simulink model "ModeAdjust"  (R2018b)
settings: Solver=FixedStepDiscrete  StartTime=0.0  StopTime=inf  FixedStep=0.01  RelTol=1e-3
undefined symbols (not defined in the file or in its folder): IfKeSMSbSeatMovBkRclnEnable_Val, IfKeSMSbSeatMovFrwdBkwdEnable_Val, IfKeSMSbSeatMovFtrstEnable_Val, IfKeSMSbSeatMovHdrstFrwdBkwdEnable_Val, IfKeSMSbSeatMovHdUpwdDnwdEnable_Val, IfKeSMSbSeatMovLgrstEnable_Val, IfKeSMSbSeatMovLtwdRtwdEnable_Val, IfVeSMSeStNumConfig, KeSMSbArmscreenMovEnable_Val, KeSMSbSeatMovLgrstExpdEnable_Val, KeSMSuFirstRwStBackPosDelta_Val, KeSMSuFirstRwStBackPosTolr_Val, KeSMSuFirstRwStCushFrntPosDelta_Val, KeSMSuFirstRwStCushFrntPosTolr_Val, KeSMSuFirstRwStCushRePosDelta_Val, KeSMSuFirstRwStCushRePosTolr_Val, KeSMSuFirstRwStFootrestPosDelta_Val, KeSMSuFirstRwStFootrestPosTolr_Val, KeSMSuFirstRwStFwdBkwdPosDelta_Val, KeSMSuFirstRwStFwdBkwdPosTolr_Val, KeSMSuMdMotFinshdTm_Val, KeSMSuMdRetryTm1_Val, KeSMSuModeReqDurgTm_Val, KeSMSuSecRwStArmTochPosDelta_Val, KeSMSuSecRwStArmTochPosTolr_Val, KeSMSuSecRwStBackPosDelta_Val, KeSMSuSecRwStBackPosTolr_Val, KeSMSuSecRwStFtrstUpwdDnwdPosDelta_Val, KeSMSuSecRwStFtrstUpwdDnwdPosTolr_Val, KeSMSuSecRwStFwdBkwdPosDelta_Val, KeSMSuSecRwStFwdBkwdPosTolr_Val, KeSMSuSecRwStHeadrestFwdBkwdPosDelta_Val, KeSMSuSecRwStHeadrestFwdBkwdPosTolr_Val, KeSMSuSecRwStHeadrestUpwdDwnwdPosDelta_Val, KeSMSuSecRwStHeadrestUpwdDwnwdPosTolr_Val, KeSMSuSecRwStLegrestInOutPosDelta_Val, KeSMSuSecRwStLegrestInOutPosTolr_Val, KeSMSuSecRwStLegrestUpwdDwnwdPosDelta_Val, KeSMSuSecRwStLegrestUpwdDwnwdPosTolr_Val, KeSMSuSecRwStLwdRwdPosDelta_Val, KeSMSuSecRwStLwdRwdPosTolr_Val, KeSMSuSecRwStVIPFtrstRefAngle_Val, KeSMSuThirdRwStFwdBkwdPosDelta_Val, KeSMSuThirdRwStFwdBkwdPosTolr_Val, KeSMSuThrdRwCushFoldPosDelta_Val, KeSMSuThrdRwCushFoldPosTolr_Val, KeSMSuThrdRwStBackPosDelta_Val, KeSMSuThrdRwStBackPosTolr_Val, KeSMSw4SLegrstCloseMdSecRwLtStFtrstUpwdDnwdPos_Val, KeSMSw4SLegrstCloseMdSecRwLtStFtrstUpwdDnwdPosMax_Val, KeSMSw4SLegrstCloseMdSecRwLtStFtrstUpwdDnwdPosMin_Val, KeSMSw4SLegrstCloseMdSecRwLtStLgrstOtwdInwdPos_Val, KeSMSw4SLegrstCloseMdSecRwLtStLgrstOtwdInwdPosMax_Val, KeSMSw4SLegrstCloseMdSecRwLtStLgrstOtwdInwdPosMin_Val, KeSMSw4SLegrstCloseMdSecRwLtStLgrstUpwdDnwdPos_Val, KeSMSw4SLegrstCloseMdSecRwLtStLgrstUpwdDnwdPosMax_Val, KeSMSw4SLegrstCloseMdSecRwLtStLgrstUpwdDnwdPosMin_Val, KeSMSw4SLegrstCloseMdSecRwRtStFtrstUpwdDnwdPos_Val, KeSMSw4SLegrstCloseMdSecRwRtStFtrstUpwdDnwdPosMax_Val, KeSMSw4SLegrstCloseMdSecRwRtStFtrstUpwdDnwdPosMin_Val ... (+1138)
libraries: Lib x401
(part 32 of 35)

== system ModeAdjust/ModeAdjustRunnable_sys/ModeAdjust/ArrivedAtTargetPosChk/VIP/R2Rt ==
  SecRwRtStPoss : Inport
  ModeStCalib_2R : Inport  Port=2
  StConfig : Inport  Port=3
  SecRwRtStPossV : Inport  Port=4
  PosDeltaCalib : Inport  Port=5
  Bus Selector : BusSelector  OutputSignals=IfVeSMSuSecRwRtStBkReclnUpwdDnwdPos_Val_read,IfVeSMSuSecRwRtStFrwdBkwdPos_Val_read,IfVeSMSuSecRwRtStHPassStUpwdDnwdPos_Val_read,IfVeSMSuSecRwRtStLgrstUpwdDnwdPos_Val_read,IfVeSMSuSecRwRtStLtwdRtwdPos_Val_read,SecRwRtStArmScrnPos_Val_read
  Bus Selector1 : BusSelector  OutputSignals=IfVeSMSuSecRwRtStBkReclnUpwdDnwdPosV_Val_read,IfVeSMSuSecRwRtStFrwdBkwdPosV_Val_read,IfVeSMSuSecRwRtStHPassStUpwdDnwdPosV_Val_read,IfVeSMSuSecRwRtStLgrstUpwdDnwdPosV_Val_read,IfVeSMSuSecRwRtStLtwdRtwdPosV_Val_read,SecRwRtStArmScrnPosV_Val_read
  Bus Selector2 : BusSelector  OutputSignals=ArmScrnPos,ArmScrnPosMax,ArmScrnPosMin,BkReclnUpwdDnwdPos,BkReclnUpwdDnwdPosMax,BkReclnUpwdDnwdPosMin,FrwdBkwdPos,FrwdBkwdPosMax,FrwdBkwdPosMin,HdrstUpwdPos,HdrstUpwdPosMax,HdrstUpwdPosMin,LgrstUpwdPos,LgrstUpwdPosMax,LgrstUpwdPosMin,LtwdRtwdPos,LtwdRtwdPosMax,LtwdRtwdPosMin
  Bus Selector3 : BusSelector  OutputSignals=VIPSecRwRtSt
  Bus Selector4 : BusSelector  OutputSignals=BkReclnUpwdDnwdMovConfig,ArmTouchMovConfig,FrwdBkwdMovConfig,LgrstUpwdMovConfig,LtwdRtwdMovConfig
  Bus Selector5 : BusSelector  OutputSignals=KeSMSuSecRwStArmTochPosDelta_Val,KeSMSuSecRwStBackPosDelta_Val,KeSMSuSecRwStFwdBkwdPosDelta_Val,KeSMSuSecRwStLegrestUpwdDwnwdPosDelta_Val,KeSMSuSecRwStLwdRwdPosDelta_Val
  CheckAtPos{,1..3} (4 alike) : Lib/CheckAtPos  SystemSampleTime=-1
  Constant{1..8} (8 alike) : Constant  Value=0  OutDataTypeStr=boolean
  IsArrivedTarZone{,1,3..4} (4 alike) : Lib/CommonUsed/IniPosjudg/Subsystem2  SystemSampleTime=-1
  Logical Operator9 : Logic  Inputs=4  AllPortsSameDT=off  OutDataTypeStr=boolean
  R2Rt_ArrivedTarPos : Outport
  wires:
  Logical Operator9/1 -> R2Rt_ArrivedTarPos/1
  IsArrivedTarZone4/1 -> [Step2_2_ArrivedTarPos]
  [SecRwRtStLtwdRtwdPos] -> IsArrivedTarZone4/1
  Bus Selector/2 -> [SecRwRtStFrwdBkwdPos]  "<IfVeSMSuSecRwRtStFrwdBkwdPos_Val_read>"
  Bus Selector/3 -> [SecRwRtStHPassStUpwdDnwdPos]  "<IfVeSMSuSecRwRtStHPassStUpwdDnwdPos_Val_read>"
  SecRwRtStPoss/1 -> Bus Selector/1
  Bus Selector/5 -> [SecRwRtStLtwdRtwdPos]  "<IfVeSMSuSecRwRtStLtwdRtwdPos_Val_read>"
  Bus Selector/1 -> [SecRwRtStBkReclnUpwdDnwdPos]  "<IfVeSMSuSecRwRtStBkReclnUpwdDnwdPos_Val_read>"
  Bus Selector/4 -> [SecRwRtStLgrstUpwdDnwdPos]  "<IfVeSMSuSecRwRtStLgrstUpwdDnwdPos_Val_read>"
  [SecRwRtStFrwdBkwdPos] -> IsArrivedTarZone3/1
  IsArrivedTarZone3/1 -> [Step2_1_ArrivedTarPos]
  IsArrivedTarZone/1 -> [Step1_1_ArrivedTarPos]
  [SecRwRtStBkReclnUpwdDnwdPos] -> IsArrivedTarZone/1
  [K_BkReclnUpwdDnwdPosMin] -> IsArrivedTarZone/2
  [K_FrwdBkwdPosMin] -> IsArrivedTarZone3/2
  [K_LgrstUpwdPosMin] -> IsArrivedTarZone1/2
  [SecRwRtStLgrstUpwdDnwdPos] -> IsArrivedTarZone1/1
  IsArrivedTarZone1/1 -> [Step1_2_ArrivedTarPos]
  Bus Selector/6 -> [SecRwRtStArmScrnPos]  "<SecRwRtStArmScrnPos_Val_read>"
  [K_LtwdRtwdPosMin] -> IsArrivedTarZone4/2
  [KeSMSuSecRwStBackPosDelta_Val] -> IsArrivedTarZone/3
  [KeSMSuSecRwStLegrestUpwdDwnwdPosDelta_Val] -> IsArrivedTarZone1/3
  [KeSMSuSecRwStFwdBkwdPosDelta_Val] -> IsArrivedTarZone3/3
  [KeSMSuSecRwStLwdRwdPosDelta_Val] -> IsArrivedTarZone4/3
  [K_BkReclnUpwdDnwdPosMax] -> IsArrivedTarZone/4
  [K_LgrstUpwdPosMax] -> IsArrivedTarZone1/4
  [K_FrwdBkwdPosMax] -> IsArrivedTarZone3/4
  [K_LtwdRtwdPosMax] -> IsArrivedTarZone4/4
  Bus Selector2/1 -> [K_ArmScrnPos]  "<ArmScrnPos>"
  Bus Selector2/18 -> [K_LtwdRtwdPosMin]  "<LtwdRtwdPosMin>"
  Bus Selector2/16 -> [K_LtwdRtwdPos]  "<LtwdRtwdPos>"
  Bus Selector2/15 -> [K_LgrstUpwdPosMin]  "<LgrstUpwdPosMin>"
  Bus Selector2/17 -> [K_LtwdRtwdPosMax]  "<LtwdRtwdPosMax>"
  Bus Selector2/12 -> [K_HdrstUpwdPosMin]  "<HdrstUpwdPosMin>"
  Bus Selector2/13 -> [K_LgrstUpwdPos]  "<LgrstUpwdPos>"
  Bus Selector2/11 -> [K_HdrstUpwdPosMax]  "<HdrstUpwdPosMax>"
  Bus Selector2/14 -> [K_LgrstUpwdPosMax]  "<LgrstUpwdPosMax>"
  Bus Selector2/10 -> [K_HdrstUpwdPos]  "<HdrstUpwdPos>"
  Bus Selector2/4 -> [K_BkReclnUpwdDnwdPos]  "<BkReclnUpwdDnwdPos>"
  Bus Selector2/9 -> [K_FrwdBkwdPosMin]  "<FrwdBkwdPosMin>"
  Bus Selector2/5 -> [K_BkReclnUpwdDnwdPosMax]  "<BkReclnUpwdDnwdPosMax>"
  Bus Selector2/8 -> [K_FrwdBkwdPosMax]  "<FrwdBkwdPosMax>"
  Bus Selector3/1 -> Bus Selector2/1  "<VIPSecRwRtSt>"
  Bus Selector2/7 -> [K_FrwdBkwdPos]  "<FrwdBkwdPos>"
  Bus Selector2/3 -> [K_ArmScrnPosMin]  "<ArmScrnPosMin>"
  Bus Selector2/2 -> [K_ArmScrnPosMax]  "<ArmScrnPosMax>"
  Bus Selector2/6 -> [K_BkReclnUpwdDnwdPosMin]  "<BkReclnUpwdDnwdPosMin>"
  ModeStCalib_2R/1 -> Bus Selector3/1
  StConfig/1 -> Bus Selector4/1
  Bus Selector4/3 -> [FrwdBkwdMovConfig]  "<FrwdBkwdMovConfig>"
  Bus Selector4/5 -> [LtwdRtwdMovConfig]  "<LtwdRtwdMovConfig>"
  Bus Selector4/4 -> [LgrstUpwdMovConfig]  "<LgrstUpwdMovConfig>"
  Bus Selector4/2 -> [ArmTouchMovConfig]  "<ArmTouchMovConfig>"
  Bus Selector4/1 -> [BkReclnUpwdDnwdMovConfig]  "<BkReclnUpwdDnwdMovConfig>"
  Bus Selector1/1 -> [SecRwRtStBkReclnUpwdDnwdPosV]  "<IfVeSMSuSecRwRtStBkReclnUpwdDnwdPosV_Val_read>"
  Bus Selector1/5 -> [SecRwRtStLtwdRtwdPosV]  "<IfVeSMSuSecRwRtStLtwdRtwdPosV_Val_read>"
  Bus Selector1/4 -> [SecRwRtStLgrstUpwdDnwdPosV]  "<IfVeSMSuSecRwRtStLgrstUpwdDnwdPosV_Val_read>"
  Bus Selector1/6 -> [SecRwRtStArmScrnPosV]  "<SecRwRtStArmScrnPosV_Val_read>"
  SecRwRtStPossV/1 -> Bus Selector1/1
  Bus Selector1/3 -> [SecRwRtStHPassStUpwdDnwdPosV]  "<IfVeSMSuSecRwRtStHPassStUpwdDnwdPosV_Val_read>"
  Bus Selector1/2 -> [SecRwRtStFrwdBkwdPosV]  "<IfVeSMSuSecRwRtStFrwdBkwdPosV_Val_read>"
  CheckAtPos2/1 -> Logical Operator9/3  "VIPR_Step2_1_ArrivedTarPos"
  CheckAtPos3/1 -> Logical Operator9/4  "VIPR_Step2_2_ArrivedTarPos"
  CheckAtPos1/1 -> Logical Operator9/2  "VIPR_Step1_2_ArrivedTarPos"
  CheckAtPos/1 -> Logical Operator9/1  "VIPR_Step1_1_ArrivedTarPos"
  [BkReclnUpwdDnwdMovConfig] -> CheckAtPos/1
  [Step1_1_ArrivedTarPos] -> CheckAtPos/3
  [LgrstUpwdMovConfig] -> CheckAtPos1/1
  [Step1_2_ArrivedTarPos] -> CheckAtPos1/3
  [FrwdBkwdMovConfig] -> CheckAtPos2/1
  [Step2_1_ArrivedTarPos] -> CheckAtPos2/3
  [LtwdRtwdMovConfig] -> CheckAtPos3/1
  [Step2_2_ArrivedTarPos] -> CheckAtPos3/3
  [SecRwRtStBkReclnUpwdDnwdPosV] -> CheckAtPos/2
  [SecRwRtStFrwdBkwdPosV] -> CheckAtPos2/2
  [SecRwRtStLgrstUpwdDnwdPosV] -> CheckAtPos1/2
  [SecRwRtStLtwdRtwdPosV] -> CheckAtPos3/2
  Constant3/1 -> CheckAtPos3/5
  Constant2/1 -> CheckAtPos3/4
  Constant4/1 -> CheckAtPos2/5
  Constant1/1 -> CheckAtPos2/4
  Constant6/1 -> CheckAtPos1/5
  Constant5/1 -> CheckAtPos1/4
  Constant8/1 -> CheckAtPos/5
  Constant7/1 -> CheckAtPos/4
  Bus Selector5/5 -> [KeSMSuSecRwStLwdRwdPosDelta_Val]  "<KeSMSuSecRwStLwdRwdPosDelta_Val>"
  PosDeltaCalib/1 -> Bus Selector5/1
  Bus Selector5/2 -> [KeSMSuSecRwStBackPosDelta_Val]  "<KeSMSuSecRwStBackPosDelta_Val>"
  Bus Selector5/4 -> [KeSMSuSecRwStLegrestUpwdDwnwdPosDelta_Val]  "<KeSMSuSecRwStLegrestUpwdDwnwdPosDelta_Val>"
  Bus Selector5/1 -> [KeSMSuSecRwStArmTochPosDelta_Val]  "<KeSMSuSecRwStArmTochPosDelta_Val>"
  Bus Selector5/3 -> [KeSMSuSecRwStFwdBkwdPosDelta_Val]  "<KeSMSuSecRwStFwdBkwdPosDelta_Val>"

== system ModeAdjust/ModeAdjustRunnable_sys/ModeAdjust/ArrivedAtTargetPosChk/VIP/R3Lt ==
  ThdRwLtStPoss : Inport
  ModeStCalib_3L : Inport  Port=2
  StConfig : Inport  Port=3
  ThdRwLtStPossV : Inport  Port=4
  PosDeltaCalib : Inport  Port=5
  Bus Selector : BusSelector  OutputSignals=IfVeSMSuThdRwLtStBkReclnUpwdDnwdPos_Val_read,IfVeSMSuThdRwLtStCshnFldUpwdDnwdPos_Val_read,IfVeSMSuThdRwLtStFrwdBkwdPos_Val_read
  Bus Selector1 : BusSelector  OutputSignals=IfVeSMSuThdRwLtStBkReclnUpwdDnwdPosV_Val_read,IfVeSMSuThdRwLtStCshnFldUpwdDnwdPosV_Val_read,IfVeSMSuThdRwLtStFrwdBkwdPosV_Val_read
  Bus Selector2 : BusSelector  OutputSignals=BkReclnUpwdDnwdPos,BkReclnUpwdDnwdPosMax,BkReclnUpwdDnwdPosMin,CshnFldUpwdDnwdPos,CshnFldUpwdDnwdPosMax,CshnFldUpwdDnwdPosMin,FrwdBkwdPos,FrwdBkwdPosMax,FrwdBkwdPosMin
  Bus Selector3 : BusSelector  OutputSignals=VIPThdRwLtSt
  Bus Selector4 : BusSelector  OutputSignals=BkReclnUpwdDnwdMovConfig,CshnFldUpwdDnwdMovConfig,FrwdBkwdMovConfig
  Bus Selector5 : BusSelector  OutputSignals=KeSMSuThirdRwStFwdBkwdPosDelta_Val,KeSMSuThrdRwCushFoldPosDelta_Val,KeSMSuThrdRwStBackPosDelta_Val
  CheckAtPos : Lib/CheckAtPos  SystemSampleTime=-1
  CheckAtPos1 : Lib/CheckAtPos  SystemSampleTime=-1
  Constant{1..4} (4 alike) : Constant  Value=0  OutDataTypeStr=boolean
  IsArrivedTarZone : Lib/CommonUsed/IniPosjudg/Subsystem2  SystemSampleTime=-1
  IsArrivedTarZone1 : Lib/CommonUsed/IniPosjudg/Subsystem2  SystemSampleTime=-1
  Logical Operator3 : Logic  AllPortsSameDT=off  OutDataTypeStr=boolean
  R3Lt_ArrivedTarPos : Outport
  wires:
  Logical Operator3/1 -> R3Lt_ArrivedTarPos/1
  Bus Selector/1 -> [ThdRwLtStBkReclnUpwdDnwdPos]  "<IfVeSMSuThdRwLtStBkReclnUpwdDnwdPos_Val_read>"
  Bus Selector/3 -> [ThdRwLtStFrwdBkwdPos]  "<IfVeSMSuThdRwLtStFrwdBkwdPos_Val_read>"
  ThdRwLtStPoss/1 -> Bus Selector/1
  Bus Selector/2 -> [ThdRwLtStCshnFldUpwdDnwdPos]  "<IfVeSMSuThdRwLtStCshnFldUpwdDnwdPos_Val_read>"
  [ThdRwLtStFrwdBkwdPos] -> IsArrivedTarZone1/1
  IsArrivedTarZone1/1 -> [Step2ArrivedTarPos]
  IsArrivedTarZone/1 -> [Step1ArrivedTarPos]
  [ThdRwLtStBkReclnUpwdDnwdPos] -> IsArrivedTarZone/1
  [K_BkReclnUpwdDnwdPosMin] -> IsArrivedTarZone/2
  [K_FrwdBkwdPosMin] -> IsArrivedTarZone1/2
  [K_BkReclnUpwdDnwdPosMax] -> IsArrivedTarZone/4
  [KeSMSuThrdRwStBackPosDelta_Val] -> IsArrivedTarZone/3
  [KeSMSuThirdRwStFwdBkwdPosDelta_Val] -> IsArrivedTarZone1/3
  [K_FrwdBkwdPosMax] -> IsArrivedTarZone1/4
  Bus Selector2/6 -> [K_CshnFldUpwdDnwdPosMin]  "<CshnFldUpwdDnwdPosMin>"
  Bus Selector2/4 -> [K_CshnFldUpwdDnwdPos]  "<CshnFldUpwdDnwdPos>"
  Bus Selector2/7 -> [K_FrwdBkwdPos]  "<FrwdBkwdPos>"
  Bus Selector2/5 -> [K_CshnFldUpwdDnwdPosMax]  "<CshnFldUpwdDnwdPosMax>"
  ModeStCalib_3L/1 -> Bus Selector3/1
  Bus Selector2/3 -> [K_BkReclnUpwdDnwdPosMin]  "<BkReclnUpwdDnwdPosMin>"
  Bus Selector3/1 -> Bus Selector2/1  "<VIPThdRwLtSt>"
  Bus Selector2/9 -> [K_FrwdBkwdPosMin]  "<FrwdBkwdPosMin>"
  Bus Selector2/2 -> [K_BkReclnUpwdDnwdPosMax]  "<BkReclnUpwdDnwdPosMax>"
  Bus Selector2/1 -> [K_BkReclnUpwdDnwdPos]  "<BkReclnUpwdDnwdPos>"
  Bus Selector2/8 -> [K_FrwdBkwdPosMax]  "<FrwdBkwdPosMax>"
  Bus Selector4/1 -> [BkReclnUpwdDnwdMovConfig]  "<BkReclnUpwdDnwdMovConfig>"
  StConfig/1 -> Bus Selector4/1
  Bus Selector4/2 -> [CshnFldUpwdDnwdMovConfig]  "<CshnFldUpwdDnwdMovConfig>"
  Bus Selector4/3 -> [FrwdBkwdMovConfig]  "<FrwdBkwdMovConfig>"
  ThdRwLtStPossV/1 -> Bus Selector1/1
  Bus Selector1/3 -> [ThdRwLtStFrwdBkwdPosV]  "<IfVeSMSuThdRwLtStFrwdBkwdPosV_Val_read>"
  Bus Selector1/2 -> [ThdRwLtStCshnFldUpwdDnwdPosV]  "<IfVeSMSuThdRwLtStCshnFldUpwdDnwdPosV_Val_read>"
  Bus Selector1/1 -> [ThdRwLtStBkReclnUpwdDnwdPosV]  "<IfVeSMSuThdRwLtStBkReclnUpwdDnwdPosV_Val_read>"
  CheckAtPos/1 -> Logical Operator3/1
  CheckAtPos1/1 -> Logical Operator3/2
  [BkReclnUpwdDnwdMovConfig] -> CheckAtPos/1
  [Step1ArrivedTarPos] -> CheckAtPos/3
  [FrwdBkwdMovConfig] -> CheckAtPos1/1
  [Step2ArrivedTarPos] -> CheckAtPos1/3
  [ThdRwLtStBkReclnUpwdDnwdPosV] -> CheckAtPos/2
  [ThdRwLtStFrwdBkwdPosV] -> CheckAtPos1/2
  Constant3/1 -> CheckAtPos/5
  Constant2/1 -> CheckAtPos/4
  Constant4/1 -> CheckAtPos1/5
  Constant1/1 -> CheckAtPos1/4
  PosDeltaCalib/1 -> Bus Selector5/1
  Bus Selector5/2 -> [KeSMSuThrdRwCushFoldPosDelta_Val]  "<KeSMSuThrdRwCushFoldPosDelta_Val>"
  Bus Selector5/1 -> [KeSMSuThirdRwStFwdBkwdPosDelta_Val]  "<KeSMSuThirdRwStFwdBkwdPosDelta_Val>"
  Bus Selector5/3 -> [KeSMSuThrdRwStBackPosDelta_Val]  "<KeSMSuThrdRwStBackPosDelta_Val>"

== system ModeAdjust/ModeAdjustRunnable_sys/ModeAdjust/ArrivedAtTargetPosChk/VIP/R3Rt ==
  ThdRwRtStPoss : Inport
  ModeStCalib_3R : Inport  Port=2
  StConfig : Inport  Port=3
  ThdRwRtStPossV : Inport  Port=4
  PosDeltaCalib : Inport  Port=5
  Bus Selector : BusSelector  OutputSignals=IfVeSMSuThdRwRtStBkReclnUpwdDnwdPos_Val_read,IfVeSMSuThdRwRtStCshnFldUpwdDnwdPos_Val_read,IfVeSMSuThdRwRtStFrwdBkwdPos_Val_read
  Bus Selector1 : BusSelector  OutputSignals=IfVeSMSuThdRwRtStBkReclnUpwdDnwdPosV_Val_read,IfVeSMSuThdRwRtStCshnFldUpwdDnwdPosV_Val_read,IfVeSMSuThdRwRtStFrwdBkwdPosV_Val_read
  Bus Selector2 : BusSelector  OutputSignals=BkReclnUpwdDnwdPos,BkReclnUpwdDnwdPosMax,BkReclnUpwdDnwdPosMin,CshnFldUpwdDnwdPos,CshnFldUpwdDnwdPosMax,CshnFldUpwdDnwdPosMin,FrwdBkwdPos,FrwdBkwdPosMax,FrwdBkwdPosMin
  Bus Selector3 : BusSelector  OutputSignals=VIPThdRwRtSt
  Bus Selector4 : BusSelector  OutputSignals=BkReclnUpwdDnwdMovConfig,CshnFldUpwdDnwdMovConfig,FrwdBkwdMovConfig
  Bus Selector5 : BusSelector  OutputSignals=KeSMSuThirdRwStFwdBkwdPosDelta_Val,KeSMSuThrdRwCushFoldPosDelta_Val,KeSMSuThrdRwStBackPosDelta_Val
  CheckAtPos : Lib/CheckAtPos  SystemSampleTime=-1
  CheckAtPos1 : Lib/CheckAtPos  SystemSampleTime=-1
  Constant{1..4} (4 alike) : Constant  Value=0  OutDataTypeStr=boolean
  IsArrivedTarZone : Lib/CommonUsed/IniPosjudg/Subsystem2  SystemSampleTime=-1
  IsArrivedTarZone1 : Lib/CommonUsed/IniPosjudg/Subsystem2  SystemSampleTime=-1
  Logical Operator3 : Logic  AllPortsSameDT=off  OutDataTypeStr=boolean
  R3Rt_ArrivedTarPos : Outport
  wires:
  Logical Operator3/1 -> R3Rt_ArrivedTarPos/1
  Bus Selector/1 -> [ThdRwRtStBkReclnUpwdDnwdPos]  "<IfVeSMSuThdRwRtStBkReclnUpwdDnwdPos_Val_read>"
  Bus Selector/2 -> [ThdRwRtStCshnFldUpwdDnwdPos]  "<IfVeSMSuThdRwRtStCshnFldUpwdDnwdPos_Val_read>"
  ThdRwRtStPoss/1 -> Bus Selector/1
  Bus Selector/3 -> [ThdRwRtStFrwdBkwdPos]  "<IfVeSMSuThdRwRtStFrwdBkwdPos_Val_read>"
  [K_FrwdBkwdPosMin] -> IsArrivedTarZone1/2
  [K_BkReclnUpwdDnwdPosMin] -> IsArrivedTarZone/2
  [ThdRwRtStBkReclnUpwdDnwdPos] -> IsArrivedTarZone/1
  IsArrivedTarZone/1 -> [Step1ArrivedTarPos]
  IsArrivedTarZone1/1 -> [Step2ArrivedTarPos]
  [ThdRwRtStFrwdBkwdPos] -> IsArrivedTarZone1/1
  [KeSMSuThrdRwStBackPosDelta_Val] -> IsArrivedTarZone/3
  [KeSMSuThirdRwStFwdBkwdPosDelta_Val] -> IsArrivedTarZone1/3
  [K_BkReclnUpwdDnwdPosMax] -> IsArrivedTarZone/4
  [K_FrwdBkwdPosMax] -> IsArrivedTarZone1/4
  Bus Selector2/6 -> [K_CshnFldUpwdDnwdPosMin]  "<CshnFldUpwdDnwdPosMin>"
  Bus Selector2/4 -> [K_CshnFldUpwdDnwdPos]  "<CshnFldUpwdDnwdPos>"
  Bus Selector2/7 -> [K_FrwdBkwdPos]  "<FrwdBkwdPos>"
  Bus Selector2/5 -> [K_CshnFldUpwdDnwdPosMax]  "<CshnFldUpwdDnwdPosMax>"
  ModeStCalib_3R/1 -> Bus Selector3/1
  Bus Selector2/3 -> [K_BkReclnUpwdDnwdPosMin]  "<BkReclnUpwdDnwdPosMin>"
  Bus Selector3/1 -> Bus Selector2/1  "<VIPThdRwRtSt>"
  Bus Selector2/9 -> [K_FrwdBkwdPosMin]  "<FrwdBkwdPosMin>"
  Bus Selector2/2 -> [K_BkReclnUpwdDnwdPosMax]  "<BkReclnUpwdDnwdPosMax>"
  Bus Selector2/1 -> [K_BkReclnUpwdDnwdPos]  "<BkReclnUpwdDnwdPos>"
  Bus Selector2/8 -> [K_FrwdBkwdPosMax]  "<FrwdBkwdPosMax>"
  Bus Selector4/1 -> [BkReclnUpwdDnwdMovConfig]  "<BkReclnUpwdDnwdMovConfig>"
  StConfig/1 -> Bus Selector4/1
  Bus Selector4/2 -> [CshnFldUpwdDnwdMovConfig]  "<CshnFldUpwdDnwdMovConfig>"
  Bus Selector4/3 -> [FrwdBkwdMovConfig]  "<FrwdBkwdMovConfig>"
  ThdRwRtStPossV/1 -> Bus Selector1/1
  Bus Selector1/1 -> [ThdRwRtStBkReclnUpwdDnwdPosV]  "<IfVeSMSuThdRwRtStBkReclnUpwdDnwdPosV_Val_read>"
  Bus Selector1/3 -> [ThdRwRtStFrwdBkwdPosV]  "<IfVeSMSuThdRwRtStFrwdBkwdPosV_Val_read>"
  Bus Selector1/2 -> [ThdRwRtStCshnFldUpwdDnwdPosV]  "<IfVeSMSuThdRwRtStCshnFldUpwdDnwdPosV_Val_read>"
  CheckAtPos/1 -> Logical Operator3/1
  CheckAtPos1/1 -> Logical Operator3/2
  [BkReclnUpwdDnwdMovConfig] -> CheckAtPos/1
  [Step1ArrivedTarPos] -> CheckAtPos/3
  [FrwdBkwdMovConfig] -> CheckAtPos1/1
  [Step2ArrivedTarPos] -> CheckAtPos1/3
  [ThdRwRtStBkReclnUpwdDnwdPosV] -> CheckAtPos/2
  [ThdRwRtStFrwdBkwdPosV] -> CheckAtPos1/2
  Constant2/1 -> CheckAtPos/4
  Constant3/1 -> CheckAtPos/5
  Constant1/1 -> CheckAtPos1/4
  Constant4/1 -> CheckAtPos1/5
  Bus Selector5/1 -> [KeSMSuThirdRwStFwdBkwdPosDelta_Val]  "<KeSMSuThirdRwStFwdBkwdPosDelta_Val>"
  Bus Selector5/2 -> [KeSMSuThrdRwCushFoldPosDelta_Val]  "<KeSMSuThrdRwCushFoldPosDelta_Val>"
  Bus Selector5/3 -> [KeSMSuThrdRwStBackPosDelta_Val]  "<KeSMSuThrdRwStBackPosDelta_Val>"
  PosDeltaCalib/1 -> Bus Selector5/1

== system ModeAdjust/ModeAdjustRunnable_sys/ModeAdjust/ArrivedAtTargetPosChk/Vip4s/R2Lt ==
  SecRwLtStsPoss : Inport
  ModeStCalib_2L : Inport  Port=2
  StConfig : Inport  Port=3
  SecRwLtStsPoss4s : Inport  Port=4
  StConfig4s : Inport  Port=5
  SecRwLtStPossV : Inport  Port=6
  SecRwLtStPossV4s : Inport  Port=7
  Lt4sHightIndex : Inport  Port=8
  PosDeltaCalib : Inport  Port=9
  Bus Creator{,1..6} (7 alike) : BusCreator  Inputs=9
  Bus Selector : BusSelector  OutputSignals=IfVeSMSuSecRwLtStBkReclnUpwdDnwdPos_Val_read,IfVeSMSuSecRwLtStFrwdBkwdPos_Val_read,IfVeSMSuSecRwLtStHPassStUpwdDnwdPos_Val_read,IfVeSMSuSecRwLtStLgrstUpwdDnwdPos_Val_read,IfVeSMSuSecRwLtStLtwdRtwdPos_Val_read,IfVeSMSuSecRwLtStArmScrnPos_Val_read
  Bus Selector1 : BusSelector  OutputSignals=IfVeSMSuSecRwLtStLgrstOtwdInwdPos_Val_read,IfVeSMSuRrLtStFtUpwdDnwdPos_Val_read,IfVeSMSuSecRwLtStHdrstFrwdBkwdPos_Val_read
  Bus Selector2 : BusSelector  OutputSignals=BkReclnUpwdDnwdPos,BkReclnUpwdDnwdPosMax,BkReclnUpwdDnwdPosMin,LgrstUpwdPos,LgrstUpwdPosMax,LgrstUpwdPosMin,FtrstUpwdDnwdPos,FtrstUpwdDnwdPosMax,FtrstUpwdDnwdPosMin
  Bus Selector3 : BusSelector  OutputSignals=VipLSecRwLtSt
  Bus Selector4 : BusSelector  OutputSignals=BkReclnUpwdDnwdMovConfig,ArmTouchMovConfig,FrwdBkwdMovConfig,LgrstUpwdMovConfig,LtwdRtwdMovConfig
  Bus Selector5 : BusSelector  OutputSignals=LgrstExpdMovConfig,FtrstMovConfig,HdrstUpwdDnwdMovConfig,HdrstFrwdBkwdMovConfig
  Bus Selector6 : BusSelector  OutputSignals=IfVeSMSuSecRwLtStBkReclnUpwdDnwdPosV_Val_read,IfVeSMSuSecRwLtStFrwdBkwdPosV_Val_read,IfVeSMSuSecRwLtStHPassStUpwdDnwdPosV_Val_read,IfVeSMSuSecRwLtStLgrstUpwdDnwdPosV_Val_read,IfVeSMSuSecRwLtStLtwdRtwdPosV_Val_read,IfVeSMSuSecRwLtStArmScrnPosV_Val_read
  Bus Selector7 : BusSelector  OutputSignals=IfVeSMSuSecRwLtStLgrstOtwdInwdPosV_Val_read,IfVeSMSuRrLtStFtUpwdDnwdPosV_Val_read,IfVeSMSuSecRwLtStHdrstFrwdBkwdPosV_Val_read
  Bus Selector8 : BusSelector  OutputSignals=HdrstUpwdDnwdPosMax,HdrstUpwdDnwdPosMin,LgrstOtwdInwdPosMax,LgrstOtwdInwdPosMin,HdrstFrwdBkwdnwdPosMax,HdrstFrwdBkwdnwdPosMin
  Bus Selector9 : BusSelector  OutputSignals=KeSMSuSecRwStHeadrestFwdBkwdPosDelta_Val,KeSMSuSecRwStHeadrestUpwdDwnwdPosDelta_Val,KeSMSuSecRwStLegrestInOutPosDelta_Val,KeSMSuSecRwStFtrstUpwdDnwdPosDelta_Val,KeSMSuSecRwStBackPosDelta_Val,KeSMSuSecRwStLegrestUpwdDwnwdPosDelta_Val
  CheckAtPos{,1..5} (6 alike) : Lib/CheckAtPos  SystemSampleTime=-1
  Constant{1..12} (12 alike) : Constant  Value=0  OutDataTypeStr=boolean
  IsArrivedTarZone{,1..5} (6 alike) : Lib/CommonUsed/IniPosjudg/Subsystem2  SystemSampleTime=-1
  Logical Operator9 : Logic  Inputs=6  AllPortsSameDT=off  OutDataTypeStr=boolean
  Multiport Switch : MultiPortSwitch  DataPortOrder=Zero-based contiguous  Inputs=7  DiagnosticForDefault=None  zeroidx=on
  PA_KeSMSw4sVIPMDSecRwLtStHdrstFrwdBkwdPosMax_160_Val : Constant  Value=KeSMSw4sVIPMDSecRwLtStHdrstFrwdBkwdPosMax_160_Val
  PA_KeSMSw4sVIPMDSecRwLtStHdrstFrwdBkwdPosMax_165_Val : Constant  Value=KeSMSw4sVIPMDSecRwLtStHdrstFrwdBkwdPosMax_165_Val
  PA_KeSMSw4sVIPMDSecRwLtStHdrstFrwdBkwdPosMax_170_Val : Constant  Value=KeSMSw4sVIPMDSecRwLtStHdrstFrwdBkwdPosMax_170_Val
  PA_KeSMSw4sVIPMDSecRwLtStHdrstFrwdBkwdPosMax_175_Val : Constant  Value=KeSMSw4sVIPMDSecRwLtStHdrstFrwdBkwdPosMax_175_Val
  PA_KeSMSw4sVIPMDSecRwLtStHdrstFrwdBkwdPosMax_180_Val : Constant  Value=KeSMSw4sVIPMDSecRwLtStHdrstFrwdBkwdPosMax_180_Val
  PA_KeSMSw4sVIPMDSecRwLtStHdrstFrwdBkwdPosMax_Below160_Val : Constant  Value=KeSMSw4sVIPMDSecRwLtStHdrstFrwdBkwdPosMax_Below160_Val
  PA_KeSMSw4sVIPMDSecRwLtStHdrstFrwdBkwdPosMax_Over180_Val : Constant  Value=KeSMSw4sVIPMDSecRwLtStHdrstFrwdBkwdPosMax_Over180_Val
  PA_KeSMSw4sVIPMDSecRwLtStHdrstFrwdBkwdPosMin_160_Val : Constant  Value=KeSMSw4sVIPMDSecRwLtStHdrstFrwdBkwdPosMin_160_Val
  PA_KeSMSw4sVIPMDSecRwLtStHdrstFrwdBkwdPosMin_165_Val : Constant  Value=KeSMSw4sVIPMDSecRwLtStHdrstFrwdBkwdPosMin_165_Val
  PA_KeSMSw4sVIPMDSecRwLtStHdrstFrwdBkwdPosMin_170_Val : Constant  Value=KeSMSw4sVIPMDSecRwLtStHdrstFrwdBkwdPosMin_170_Val
  PA_KeSMSw4sVIPMDSecRwLtStHdrstFrwdBkwdPosMin_175_Val : Constant  Value=KeSMSw4sVIPMDSecRwLtStHdrstFrwdBkwdPosMin_175_Val
  PA_KeSMSw4sVIPMDSecRwLtStHdrstFrwdBkwdPosMin_180_Val : Constant  Value=KeSMSw4sVIPMDSecRwLtStHdrstFrwdBkwdPosMin_180_Val
  PA_KeSMSw4sVIPMDSecRwLtStHdrstFrwdBkwdPosMin_Below160_Val : Constant  Value=KeSMSw4sVIPMDSecRwLtStHdrstFrwdBkwdPosMin_Below160_Val
  PA_KeSMSw4sVIPMDSecRwLtStHdrstFrwdBkwdPosMin_Over180_Val : Constant  Value=KeSMSw4sVIPMDSecRwLtStHdrstFrwdBkwdPosMin_Over180_Val
  PA_KeSMSw4sVIPMDSecRwLtStHdrstFrwdBkwdPos_160_Val : Constant  Value=KeSMSw4sVIPMDSecRwLtStHdrstFrwdBkwdPos_160_Val
  PA_KeSMSw4sVIPMDSecRwLtStHdrstFrwdBkwdPos_165_Val : Constant  Value=KeSMSw4sVIPMDSecRwLtStHdrstFrwdBkwdPos_165_Val
  PA_KeSMSw4sVIPMDSecRwLtStHdrstFrwdBkwdPos_170_Val : Constant  Value=KeSMSw4sVIPMDSecRwLtStHdrstFrwdBkwdPos_170_Val
  PA_KeSMSw4sVIPMDSecRwLtStHdrstFrwdBkwdPos_175_Val : Constant  Value=KeSMSw4sVIPMDSecRwLtStHdrstFrwdBkwdPos_175_Val
  PA_KeSMSw4sVIPMDSecRwLtStHdrstFrwdBkwdPos_180_Val : Constant  Value=KeSMSw4sVIPMDSecRwLtStHdrstFrwdBkwdPos_180_Val
  PA_KeSMSw4sVIPMDSecRwLtStHdrstFrwdBkwdPos_Below160_Val : Constant  Value=KeSMSw4sVIPMDSecRwLtStHdrstFrwdBkwdPos_Below160_Val
  PA_KeSMSw4sVIPMDSecRwLtStHdrstFrwdBkwdPos_Over180_Val : Constant  Value=KeSMSw4sVIPMDSecRwLtStHdrstFrwdBkwdPos_Over180_Val
  PA_KeSMSw4sVIPMDSecRwLtStHdrstUpwdDnwdPosMax_160_Val : Constant  Value=KeSMSw4sVIPMDSecRwLtStHdrstUpwdDnwdPosMax_160_Val
  PA_KeSMSw4sVIPMDSecRwLtStHdrstUpwdDnwdPosMax_165_Val : Constant  Value=KeSMSw4sVIPMDSecRwLtStHdrstUpwdDnwdPosMax_165_Val
  PA_KeSMSw4sVIPMDSecRwLtStHdrstUpwdDnwdPosMax_170_Val : Constant  Value=KeSMSw4sVIPMDSecRwLtStHdrstUpwdDnwdPosMax_170_Val
  PA_KeSMSw4sVIPMDSecRwLtStHdrstUpwdDnwdPosMax_175_Val : Constant  Value=KeSMSw4sVIPMDSecRwLtStHdrstUpwdDnwdPosMax_175_Val
  PA_KeSMSw4sVIPMDSecRwLtStHdrstUpwdDnwdPosMax_180_Val : Constant  Value=KeSMSw4sVIPMDSecRwLtStHdrstUpwdDnwdPosMax_180_Val
  PA_KeSMSw4sVIPMDSecRwLtStHdrstUpwdDnwdPosMax_Below160_Val : Constant  Value=KeSMSw4sVIPMDSecRwLtStHdrstUpwdDnwdPosMax_Below160_Val
  PA_KeSMSw4sVIPMDSecRwLtStHdrstUpwdDnwdPosMax_Over180_Val : Constant  Value=KeSMSw4sVIPMDSecRwLtStHdrstUpwdDnwdPosMax_Over180_Val
  PA_KeSMSw4sVIPMDSecRwLtStHdrstUpwdDnwdPosMin_160_Val : Constant  Value=KeSMSw4sVIPMDSecRwLtStHdrstUpwdDnwdPosMin_160_Val
  PA_KeSMSw4sVIPMDSecRwLtStHdrstUpwdDnwdPosMin_165_Val : Constant  Value=KeSMSw4sVIPMDSecRwLtStHdrstUpwdDnwdPosMin_165_Val
  PA_KeSMSw4sVIPMDSecRwLtStHdrstUpwdDnwdPosMin_170_Val : Constant  Value=KeSMSw4sVIPMDSecRwLtStHdrstUpwdDnwdPosMin_170_Val
  PA_KeSMSw4sVIPMDSecRwLtStHdrstUpwdDnwdPosMin_175_Val : Constant  Value=KeSMSw4sVIPMDSecRwLtStHdrstUpwdDnwdPosMin_175_Val
  PA_KeSMSw4sVIPMDSecRwLtStHdrstUpwdDnwdPosMin_180_Val : Constant  Value=KeSMSw4sVIPMDSecRwLtStHdrstUpwdDnwdPosMin_180_Val
  PA_KeSMSw4sVIPMDSecRwLtStHdrstUpwdDnwdPosMin_Below160_Val : Constant  Value=KeSMSw4sVIPMDSecRwLtStHdrstUpwdDnwdPosMin_Below160_Val
  PA_KeSMSw4sVIPMDSecRwLtStHdrstUpwdDnwdPosMin_Over180_Val : Constant  Value=KeSMSw4sVIPMDSecRwLtStHdrstUpwdDnwdPosMin_Over180_Val
  PA_KeSMSw4sVIPMDSecRwLtStHdrstUpwdDnwdPos_160_Val : Constant  Value=KeSMSw4sVIPMDSecRwLtStHdrstUpwdDnwdPos_160_Val
  PA_KeSMSw4sVIPMDSecRwLtStHdrstUpwdDnwdPos_165_Val : Constant  Value=KeSMSw4sVIPMDSecRwLtStHdrstUpwdDnwdPos_165_Val
  PA_KeSMSw4sVIPMDSecRwLtStHdrstUpwdDnwdPos_170_Val : Constant  Value=KeSMSw4sVIPMDSecRwLtStHdrstUpwdDnwdPos_170_Val
  PA_KeSMSw4sVIPMDSecRwLtStHdrstUpwdDnwdPos_175_Val : Constant  Value=KeSMSw4sVIPMDSecRwLtStHdrstUpwdDnwdPos_175_Val
  PA_KeSMSw4sVIPMDSecRwLtStHdrstUpwdDnwdPos_180_Val : Constant  Value=KeSMSw4sVIPMDSecRwLtStHdrstUpwdDnwdPos_180_Val
  PA_KeSMSw4sVIPMDSecRwLtStHdrstUpwdDnwdPos_Below160_Val : Constant  Value=KeSMSw4sVIPMDSecRwLtStHdrstUpwdDnwdPos_Below160_Val
  PA_KeSMSw4sVIPMDSecRwLtStHdrstUpwdDnwdPos_Over180_Val : Constant  Value=KeSMSw4sVIPMDSecRwLtStHdrstUpwdDnwdPos_Over180_Val
  PA_KeSMSw4sVIPMDSecRwLtStLgrstOtwdInwdPosMax_160_Val : Constant  Value=KeSMSw4sVIPMDSecRwLtStLgrstOtwdInwdPosMax_160_Val
  PA_KeSMSw4sVIPMDSecRwLtStLgrstOtwdInwdPosMax_165_Val : Constant  Value=KeSMSw4sVIPMDSecRwLtStLgrstOtwdInwdPosMax_165_Val
  PA_KeSMSw4sVIPMDSecRwLtStLgrstOtwdInwdPosMax_170_Val : Constant  Value=KeSMSw4sVIPMDSecRwLtStLgrstOtwdInwdPosMax_170_Val
  PA_KeSMSw4sVIPMDSecRwLtStLgrstOtwdInwdPosMax_175_Val : Constant  Value=KeSMSw4sVIPMDSecRwLtStLgrstOtwdInwdPosMax_175_Val
  PA_KeSMSw4sVIPMDSecRwLtStLgrstOtwdInwdPosMax_180_Val : Constant  Value=KeSMSw4sVIPMDSecRwLtStLgrstOtwdInwdPosMax_180_Val
  PA_KeSMSw4sVIPMDSecRwLtStLgrstOtwdInwdPosMax_Below160_Val : Constant  Value=KeSMSw4sVIPMDSecRwLtStLgrstOtwdInwdPosMax_Below160_Val
  PA_KeSMSw4sVIPMDSecRwLtStLgrstOtwdInwdPosMax_Over180_Val : Constant  Value=KeSMSw4sVIPMDSecRwLtStLgrstOtwdInwdPosMin_180_Val
  PA_KeSMSw4sVIPMDSecRwLtStLgrstOtwdInwdPosMin_160_Val : Constant  Value=KeSMSw4sVIPMDSecRwLtStLgrstOtwdInwdPosMin_160_Val
  PA_KeSMSw4sVIPMDSecRwLtStLgrstOtwdInwdPosMin_165_Val : Constant  Value=KeSMSw4sVIPMDSecRwLtStLgrstOtwdInwdPosMin_165_Val
  PA_KeSMSw4sVIPMDSecRwLtStLgrstOtwdInwdPosMin_170_Val : Constant  Value=KeSMSw4sVIPMDSecRwLtStLgrstOtwdInwdPosMin_170_Val
  PA_KeSMSw4sVIPMDSecRwLtStLgrstOtwdInwdPosMin_175_Val : Constant  Value=KeSMSw4sVIPMDSecRwLtStLgrstOtwdInwdPosMin_175_Val
  PA_KeSMSw4sVIPMDSecRwLtStLgrstOtwdInwdPosMin_180_Val : Constant  Value=KeSMSw4sVIPMDSecRwLtStLgrstOtwdInwdPosMax_Over180_Val
  PA_KeSMSw4sVIPMDSecRwLtStLgrstOtwdInwdPosMin_Below160_Val : Constant  Value=KeSMSw4sVIPMDSecRwLtStLgrstOtwdInwdPosMin_Below160_Val
  PA_KeSMSw4sVIPMDSecRwLtStLgrstOtwdInwdPosMin_Over180_Val : Constant  Value=KeSMSw4sVIPMDSecRwLtStLgrstOtwdInwdPosMin_Over180_Val
  PA_KeSMSw4sVIPMDSecRwLtStLgrstOtwdInwdPos_160_Val : Constant  Value=KeSMSw4sVIPMDSecRwLtStLgrstOtwdInwdPos_160_Val
  PA_KeSMSw4sVIPMDSecRwLtStLgrstOtwdInwdPos_165_Val : Constant  Value=KeSMSw4sVIPMDSecRwLtStLgrstOtwdInwdPos_165_Val
  PA_KeSMSw4sVIPMDSecRwLtStLgrstOtwdInwdPos_170_Val : Constant  Value=KeSMSw4sVIPMDSecRwLtStLgrstOtwdInwdPos_170_Val
  PA_KeSMSw4sVIPMDSecRwLtStLgrstOtwdInwdPos_175_Val : Constant  Value=KeSMSw4sVIPMDSecRwLtStLgrstOtwdInwdPos_175_Val
  PA_KeSMSw4sVIPMDSecRwLtStLgrstOtwdInwdPos_180_Val : Constant  Value=KeSMSw4sVIPMDSecRwLtStLgrstOtwdInwdPos_180_Val
  PA_KeSMSw4sVIPMDSecRwLtStLgrstOtwdInwdPos_Below160_Val : Constant  Value=KeSMSw4sVIPMDSecRwLtStLgrstOtwdInwdPos_Below160_Val
  PA_KeSMSw4sVIPMDSecRwLtStLgrstOtwdInwdPos_Over180_Val : Constant  Value=KeSMSw4sVIPMDSecRwLtStLgrstOtwdInwdPos_Over180_Val
  R2Lt_ArrivedTarPos : Outport
  Calib_VIP4sLAdpt : Outport  Port=2
  wires:
  Bus Selector5/2 -> [FtrstMovConfig]  "<FtrstMovConfig>"
  Bus Selector5/1 -> [LgrstExpdMovConfig]  "<LgrstExpdMovConfig>"
  Bus Selector5/3 -> [HdrstMovConfig]  "<HdrstUpwdDnwdMovConfig>"
  StConfig4s/1 -> Bus Selector5/1
  IsArrivedTarZone4/1 -> [Step1_5_ArrivedTarPos]
  [KeSMSuSecRwStLegrestInOutPosDelta_Val] -> IsArrivedTarZone4/3
  [SecRwLtStLgrstOtwdInwdPos] -> IsArrivedTarZone4/1
  [K_LgrstOtwdInwdPos_Max] -> IsArrivedTarZone4/4
  [K_LgrstOtwdInwdPos_Min] -> IsArrivedTarZone4/2
  IsArrivedTarZone3/1 -> [Step1_4_ArrivedTarPos]
  [K_FtrstUpwdDnwdPos_Max] -> IsArrivedTarZone3/4
  [K_FtrstUpwdDnwdPos_Min] -> IsArrivedTarZone3/2
  Bus Selector2/9 -> [K_FtrstUpwdDnwdPos_Min]  "<FtrstUpwdDnwdPosMin>"
  Bus Selector2/8 -> [K_FtrstUpwdDnwdPos_Max]  "<FtrstUpwdDnwdPosMax>"
  Bus Selector2/7 -> [K_FtrstUpwdDnwdPos]  "<FtrstUpwdDnwdPos>"
  [IfVeSMSuRrLtStFtUpwdDnwdPos] -> IsArrivedTarZone3/1
  Bus Selector1/2 -> [IfVeSMSuRrLtStFtUpwdDnwdPos]  "<IfVeSMSuRrLtStFtUpwdDnwdPos_Val_read>"
  Bus Selector1/1 -> [SecRwLtStLgrstOtwdInwdPos]  "<IfVeSMSuSecRwLtStLgrstOtwdInwdPos_Val_read>"
  SecRwLtStsPoss4s/1 -> Bus Selector1/1
  [KeSMSuSecRwStFtrstUpwdDnwdPosDelta_Val] -> IsArrivedTarZone3/3
  [KeSMSuSecRwStHeadrestUpwdDwnwdPosDelta_Val] -> IsArrivedTarZone2/3
  [SecRwLtStHPassStUpwdDnwdPos] -> IsArrivedTarZone2/1
  [K_HdrstUpwdPosMin] -> IsArrivedTarZone2/2
  [K_HdrstUpwdPosMax] -> IsArrivedTarZone2/4
  Bus Selector4/1 -> [BkReclnUpwdDnwdMovConfig]  "<BkReclnUpwdDnwdMovConfig>"
  Bus Selector4/2 -> [ArmTouchMovConfig]  "<ArmTouchMovConfig>"
  Bus Selector4/4 -> [LgrstUpwdMovConfig]  "<LgrstUpwdMovConfig>"
  Bus Selector4/5 -> [LtwdRtwdMovConfig]  "<LtwdRtwdMovConfig>"
  Bus Selector4/3 -> [FrwdBkwdMovConfig]  "<FrwdBkwdMovConfig>"
  StConfig/1 -> Bus Selector4/1
  ModeStCalib_2L/1 -> Bus Selector3/1
  Bus Selector2/3 -> [K_BkReclnUpwdDnwdPosMin]  "<BkReclnUpwdDnwdPosMin>"
  Bus Selector3/1 -> Bus Selector2/1  "<VipLSecRwLtSt>"
  Bus Selector2/2 -> [K_BkReclnUpwdDnwdPosMax]  "<BkReclnUpwdDnwdPosMax>"
  Bus Selector2/1 -> [K_BkReclnUpwdDnwdPos]  "<BkReclnUpwdDnwdPos>"
  Bus Selector2/5 -> [K_LgrstUpwdPosMax]  "<LgrstUpwdPosMax>"
  Bus Selector2/4 -> [K_LgrstUpwdPos]  "<LgrstUpwdPos>"
  Bus Selector2/6 -> [K_LgrstUpwdPosMin]  "<LgrstUpwdPosMin>"
  [KeSMSuSecRwStLegrestUpwdDwnwdPosDelta_Val] -> IsArrivedTarZone1/3
  [K_LgrstUpwdPosMax] -> IsArrivedTarZone1/4
  [K_BkReclnUpwdDnwdPosMax] -> IsArrivedTarZone/4
  [KeSMSuSecRwStBackPosDelta_Val] -> IsArrivedTarZone/3
  Bus Selector/6 -> [SecRwLtStArmScrnPos]  "<IfVeSMSuSecRwLtStArmScrnPos_Val_read>"
  IsArrivedTarZone2/1 -> [Step1_3_ArrivedTarPos]
  Logical Operator9/1 -> R2Lt_ArrivedTarPos/1
  IsArrivedTarZone1/1 -> [Step1_2_ArrivedTarPos]
  [SecRwLtStLgrstUpwdDnwdPos] -> IsArrivedTarZone1/1
  [K_LgrstUpwdPosMin] -> IsArrivedTarZone1/2
  Bus Selector/1 -> [SecRwLtStBkReclnUpwdDnwdPos]  "<IfVeSMSuSecRwLtStBkReclnUpwdDnwdPos_Val_read>"
  Bus Selector/2 -> [SecRwLtStFrwdBkwdPos]  "<IfVeSMSuSecRwLtStFrwdBkwdPos_Val_read>"
  Bus Selector/4 -> [SecRwLtStLgrstUpwdDnwdPos]  "<IfVeSMSuSecRwLtStLgrstUpwdDnwdPos_Val_read>"
  Bus Selector/3 -> [SecRwLtStHPassStUpwdDnwdPos]  "<IfVeSMSuSecRwLtStHPassStUpwdDnwdPos_Val_read>"
  SecRwLtStsPoss/1 -> Bus Selector/1
  Bus Selector/5 -> [SecRwLtStLtwdRtwdPos]  "<IfVeSMSuSecRwLtStLtwdRtwdPos_Val_read>"
  [K_BkReclnUpwdDnwdPosMin] -> IsArrivedTarZone/2
  [SecRwLtStBkReclnUpwdDnwdPos] -> IsArrivedTarZone/1
  IsArrivedTarZone/1 -> [Step1_1_ArrivedTarPos]
  Bus Selector7/2 -> [RrLtStFtUpwdDnwdPosV]  "<IfVeSMSuRrLtStFtUpwdDnwdPosV_Val_read>"
  SecRwLtStPossV4s/1 -> Bus Selector7/1
  Bus Selector7/1 -> [SecRwLtStLgrstOtwdInwdPosV]  "<IfVeSMSuSecRwLtStLgrstOtwdInwdPosV_Val_read>"
  Bus Selector6/1 -> [SecRwLtStBkReclnUpwdDnwdPosV]  "<IfVeSMSuSecRwLtStBkReclnUpwdDnwdPosV_Val_read>"
  SecRwLtStPossV/1 -> Bus Selector6/1
  Bus Selector6/4 -> [SecRwLtStLgrstUpwdDnwdPosV]  "<IfVeSMSuSecRwLtStLgrstUpwdDnwdPosV_Val_read>"
  Bus Selector6/5 -> [SecRwLtStLtwdRtwdPosV]  "<IfVeSMSuSecRwLtStLtwdRtwdPosV_Val_read>"
  Bus Selector6/6 -> [IfVeSMSuSecRwLtStArmScrnPosV]  "<IfVeSMSuSecRwLtStArmScrnPosV_Val_read>"
  Bus Selector6/3 -> [SecRwLtStHPassStUpwdDnwdPosV]  "<IfVeSMSuSecRwLtStHPassStUpwdDnwdPosV_Val_read>"
  Bus Selector6/2 -> [SecRwLtStFrwdBkwdPosV]  "<IfVeSMSuSecRwLtStFrwdBkwdPosV_Val_read>"
  CheckAtPos2/1 -> Logical Operator9/3  "vip4sL_Step1_3_ArrivedTarPos"
  CheckAtPos1/1 -> Logical Operator9/2  "vip4sL_Step1_2_ArrivedTarPos"
  CheckAtPos3/1 -> Logical Operator9/4  "vip4sL_Step1_4_ArrivedTarPos"
  CheckAtPos/1 -> Logical Operator9/1  "vip4sL_Step1_1_ArrivedTarPos"
  CheckAtPos4/1 -> Logical Operator9/5  "vip4sL_Step1_5_ArrivedTarPos"
  [BkReclnUpwdDnwdMovConfig] -> CheckAtPos/1
  [Step1_1_ArrivedTarPos] -> CheckAtPos/3
  [LgrstUpwdMovConfig] -> CheckAtPos1/1
  [Step1_2_ArrivedTarPos] -> CheckAtPos1/3
  [HdrstMovConfig] -> CheckAtPos2/1
  [Step1_3_ArrivedTarPos] -> CheckAtPos2/3
  [FtrstMovConfig] -> CheckAtPos3/1
  [Step1_4_ArrivedTarPos] -> CheckAtPos3/3
  [LgrstExpdMovConfig] -> CheckAtPos4/1
  [Step1_5_ArrivedTarPos] -> CheckAtPos4/3
  [SecRwLtStBkReclnUpwdDnwdPosV] -> CheckAtPos/2
  [SecRwLtStLgrstUpwdDnwdPosV] -> CheckAtPos1/2
  [SecRwLtStHPassStUpwdDnwdPosV] -> CheckAtPos2/2
  [RrLtStFtUpwdDnwdPosV] -> CheckAtPos3/2
  [SecRwLtStLgrstOtwdInwdPosV] -> CheckAtPos4/2
  Constant9/1 -> CheckAtPos4/4
  Constant10/1 -> CheckAtPos4/5
  Constant2/1 -> CheckAtPos3/4
  Constant1/1 -> CheckAtPos3/5
  Constant4/1 -> CheckAtPos2/4
  Constant3/1 -> CheckAtPos2/5
  Constant6/1 -> CheckAtPos1/4
  Constant5/1 -> CheckAtPos1/5
  Constant8/1 -> CheckAtPos/4
  Constant7/1 -> CheckAtPos/5
  [SecRwLtStHdrstFrwdBkwdPos] -> IsArrivedTarZone5/1
  [K_HdrstFrwdBkwdnwdPosMin] -> IsArrivedTarZone5/2
  [HdrstFrwdBkwdMovConfig] -> CheckAtPos5/1
  Constant12/1 -> CheckAtPos5/4
  Constant11/1 -> CheckAtPos5/5
  [Step1_6_ArrivedTarPos] -> CheckAtPos5/3
  [KeSMSuSecRwStHeadrestFwdBkwdPosDelta_Val] -> IsArrivedTarZone5/3
  [K_HdrstFrwdBkwdnwdPosMax] -> IsArrivedTarZone5/4
  IsArrivedTarZone5/1 -> [Step1_6_ArrivedTarPos]
  [SecRwLtStHdrstFrwdBkwdPosV] -> CheckAtPos5/2
  CheckAtPos5/1 -> Logical Operator9/6  "vip4sL_Step1_6_ArrivedTarPos"
  Bus Selector7/3 -> [SecRwLtStHdrstFrwdBkwdPosV]  "<IfVeSMSuSecRwLtStHdrstFrwdBkwdPosV_Val_read>"
  Bus Selector5/4 -> [HdrstFrwdBkwdMovConfig]  "<HdrstFrwdBkwdMovConfig>"
  Bus Selector1/3 -> [SecRwLtStHdrstFrwdBkwdPos]  "<IfVeSMSuSecRwLtStHdrstFrwdBkwdPos_Val_read>"
  Lt4sHightIndex/1 -> Multiport Switch/1
  PA_KeSMSw4sVIPMDSecRwLtStHdrstUpwdDnwdPos_Below160_Val/1 -> Bus Creator/1  "HdrstUpwdDnwdPos"
  PA_KeSMSw4sVIPMDSecRwLtStHdrstUpwdDnwdPosMax_Below160_Val/1 -> Bus Creator/2  "HdrstUpwdDnwdPosMax"
  PA_KeSMSw4sVIPMDSecRwLtStHdrstUpwdDnwdPosMin_Below160_Val/1 -> Bus Creator/3  "HdrstUpwdDnwdPosMin"
  PA_KeSMSw4sVIPMDSecRwLtStLgrstOtwdInwdPos_Below160_Val/1 -> Bus Creator/4  "LgrstOtwdInwdPos"
  PA_KeSMSw4sVIPMDSecRwLtStLgrstOtwdInwdPosMax_Below160_Val/1 -> Bus Creator/5  "LgrstOtwdInwdPosMax"
  PA_KeSMSw4sVIPMDSecRwLtStLgrstOtwdInwdPosMin_Below160_Val/1 -> Bus Creator/6  "LgrstOtwdInwdPosMin"
  Bus Creator/1 -> Multiport Switch/2  "VIP4sLAdpt"
  Multiport Switch/1 -> Calib_VIP4sLAdpt/1, Bus Selector8/1
  Bus Selector8/2 -> [K_HdrstUpwdPosMin]  "<HdrstUpwdDnwdPosMin>"
  Bus Selector8/3 -> [K_LgrstOtwdInwdPos_Max]  "<LgrstOtwdInwdPosMax>"
  Bus Selector8/1 -> [K_HdrstUpwdPosMax]  "<HdrstUpwdDnwdPosMax>"
  Bus Selector8/4 -> [K_LgrstOtwdInwdPos_Min]  "<LgrstOtwdInwdPosMin>"
  PA_KeSMSw4sVIPMDSecRwLtStHdrstFrwdBkwdPos_Below160_Val/1 -> Bus Creator/7  "HdrstFrwdBkwdnwdPos"
  PA_KeSMSw4sVIPMDSecRwLtStHdrstFrwdBkwdPosMax_Below160_Val/1 -> Bus Creator/8  "HdrstFrwdBkwdnwdPosMax"
  PA_KeSMSw4sVIPMDSecRwLtStHdrstFrwdBkwdPosMin_Below160_Val/1 -> Bus Creator/9  "HdrstFrwdBkwdnwdPosMin"
  PA_KeSMSw4sVIPMDSecRwLtStLgrstOtwdInwdPos_160_Val/1 -> Bus Creator1/4  "LgrstOtwdInwdPos"
  PA_KeSMSw4sVIPMDSecRwLtStLgrstOtwdInwdPosMin_160_Val/1 -> Bus Creator1/6  "LgrstOtwdInwdPosMin"
  PA_KeSMSw4sVIPMDSecRwLtStHdrstUpwdDnwdPos_160_Val/1 -> Bus Creator1/1  "HdrstUpwdDnwdPos"
  PA_KeSMSw4sVIPMDSecRwLtStHdrstUpwdDnwdPosMin_160_Val/1 -> Bus Creator1/3  "HdrstUpwdDnwdPosMin"
  PA_KeSMSw4sVIPMDSecRwLtStHdrstUpwdDnwdPosMax_160_Val/1 -> Bus Creator1/2  "HdrstUpwdDnwdPosMax"
  PA_KeSMSw4sVIPMDSecRwLtStLgrstOtwdInwdPosMax_160_Val/1 -> Bus Creator1/5  "LgrstOtwdInwdPosMax"
  PA_KeSMSw4sVIPMDSecRwLtStHdrstFrwdBkwdPosMin_160_Val/1 -> Bus Creator1/9  "HdrstFrwdBkwdnwdPosMin"
  PA_KeSMSw4sVIPMDSecRwLtStHdrstFrwdBkwdPosMax_160_Val/1 -> Bus Creator1/8  "HdrstFrwdBkwdnwdPosMax"
  PA_KeSMSw4sVIPMDSecRwLtStHdrstFrwdBkwdPos_160_Val/1 -> Bus Creator1/7  "HdrstFrwdBkwdnwdPos"
  Bus Creator1/1 -> Multiport Switch/3  "VIP4sLAdpt"
  PA_KeSMSw4sVIPMDSecRwLtStLgrstOtwdInwdPos_165_Val/1 -> Bus Creator2/4  "LgrstOtwdInwdPos"
  PA_KeSMSw4sVIPMDSecRwLtStLgrstOtwdInwdPosMin_165_Val/1 -> Bus Creator2/6  "LgrstOtwdInwdPosMin"
  PA_KeSMSw4sVIPMDSecRwLtStHdrstUpwdDnwdPos_165_Val/1 -> Bus Creator2/1  "HdrstUpwdDnwdPos"
  PA_KeSMSw4sVIPMDSecRwLtStHdrstUpwdDnwdPosMin_165_Val/1 -> Bus Creator2/3  "HdrstUpwdDnwdPosMin"
  PA_KeSMSw4sVIPMDSecRwLtStHdrstUpwdDnwdPosMax_165_Val/1 -> Bus Creator2/2  "HdrstUpwdDnwdPosMax"
  PA_KeSMSw4sVIPMDSecRwLtStLgrstOtwdInwdPosMax_165_Val/1 -> Bus Creator2/5  "LgrstOtwdInwdPosMax"
  PA_KeSMSw4sVIPMDSecRwLtStHdrstFrwdBkwdPosMin_165_Val/1 -> Bus Creator2/9  "HdrstFrwdBkwdnwdPosMin"
  PA_KeSMSw4sVIPMDSecRwLtStHdrstFrwdBkwdPosMax_165_Val/1 -> Bus Creator2/8  "HdrstFrwdBkwdnwdPosMax"
  PA_KeSMSw4sVIPMDSecRwLtStHdrstFrwdBkwdPos_165_Val/1 -> Bus Creator2/7  "HdrstFrwdBkwdnwdPos"
  Bus Creator2/1 -> Multiport Switch/4  "VIP4sLAdpt"
  PA_KeSMSw4sVIPMDSecRwLtStLgrstOtwdInwdPos_170_Val/1 -> Bus Creator3/4  "LgrstOtwdInwdPos"
  PA_KeSMSw4sVIPMDSecRwLtStLgrstOtwdInwdPosMin_170_Val/1 -> Bus Creator3/6  "LgrstOtwdInwdPosMin"
  PA_KeSMSw4sVIPMDSecRwLtStHdrstUpwdDnwdPos_170_Val/1 -> Bus Creator3/1  "HdrstUpwdDnwdPos"
  PA_KeSMSw4sVIPMDSecRwLtStHdrstUpwdDnwdPosMin_170_Val/1 -> Bus Creator3/3  "HdrstUpwdDnwdPosMin"
  PA_KeSMSw4sVIPMDSecRwLtStHdrstUpwdDnwdPosMax_170_Val/1 -> Bus Creator3/2  "HdrstUpwdDnwdPosMax"
  PA_KeSMSw4sVIPMDSecRwLtStLgrstOtwdInwdPosMax_170_Val/1 -> Bus Creator3/5  "LgrstOtwdInwdPosMax"
  PA_KeSMSw4sVIPMDSecRwLtStHdrstFrwdBkwdPosMin_170_Val/1 -> Bus Creator3/9  "HdrstFrwdBkwdnwdPosMin"
  PA_KeSMSw4sVIPMDSecRwLtStHdrstFrwdBkwdPosMax_170_Val/1 -> Bus Creator3/8  "HdrstFrwdBkwdnwdPosMax"
  PA_KeSMSw4sVIPMDSecRwLtStHdrstFrwdBkwdPos_170_Val/1 -> Bus Creator3/7  "HdrstFrwdBkwdnwdPos"
  Bus Creator3/1 -> Multiport Switch/5  "VIP4sLAdpt"
  PA_KeSMSw4sVIPMDSecRwLtStLgrstOtwdInwdPos_175_Val/1 -> Bus Creator4/4  "LgrstOtwdInwdPos"
  PA_KeSMSw4sVIPMDSecRwLtStLgrstOtwdInwdPosMin_175_Val/1 -> Bus Creator4/6  "LgrstOtwdInwdPosMin"
  PA_KeSMSw4sVIPMDSecRwLtStHdrstUpwdDnwdPos_175_Val/1 -> Bus Creator4/1  "HdrstUpwdDnwdPos"
  PA_KeSMSw4sVIPMDSecRwLtStHdrstUpwdDnwdPosMin_175_Val/1 -> Bus Creator4/3  "HdrstUpwdDnwdPosMin"
  PA_KeSMSw4sVIPMDSecRwLtStHdrstUpwdDnwdPosMax_175_Val/1 -> Bus Creator4/2  "HdrstUpwdDnwdPosMax"
  PA_KeSMSw4sVIPMDSecRwLtStLgrstOtwdInwdPosMax_175_Val/1 -> Bus Creator4/5  "LgrstOtwdInwdPosMax"
  PA_KeSMSw4sVIPMDSecRwLtStHdrstFrwdBkwdPosMin_175_Val/1 -> Bus Creator4/9  "HdrstFrwdBkwdnwdPosMin"
  PA_KeSMSw4sVIPMDSecRwLtStHdrstFrwdBkwdPosMax_175_Val/1 -> Bus Creator4/8  "HdrstFrwdBkwdnwdPosMax"
  PA_KeSMSw4sVIPMDSecRwLtStHdrstFrwdBkwdPos_175_Val/1 -> Bus Creator4/7  "HdrstFrwdBkwdnwdPos"
  Bus Creator4/1 -> Multiport Switch/6  "VIP4sLAdpt"
  PA_KeSMSw4sVIPMDSecRwLtStLgrstOtwdInwdPos_180_Val/1 -> Bus Creator5/4  "LgrstOtwdInwdPos"
  PA_KeSMSw4sVIPMDSecRwLtStLgrstOtwdInwdPosMax_Over180_Val/1 -> Bus Creator5/6  "LgrstOtwdInwdPosMin"
  PA_KeSMSw4sVIPMDSecRwLtStHdrstUpwdDnwdPos_180_Val/1 -> Bus Creator5/1  "HdrstUpwdDnwdPos"
  PA_KeSMSw4sVIPMDSecRwLtStHdrstUpwdDnwdPosMin_180_Val/1 -> Bus Creator5/3  "HdrstUpwdDnwdPosMin"
  PA_KeSMSw4sVIPMDSecRwLtStHdrstUpwdDnwdPosMax_180_Val/1 -> Bus Creator5/2  "HdrstUpwdDnwdPosMax"
  PA_KeSMSw4sVIPMDSecRwLtStLgrstOtwdInwdPosMax_180_Val/1 -> Bus Creator5/5  "LgrstOtwdInwdPosMax"
  PA_KeSMSw4sVIPMDSecRwLtStHdrstFrwdBkwdPosMin_180_Val/1 -> Bus Creator5/9  "HdrstFrwdBkwdnwdPosMin"
  PA_KeSMSw4sVIPMDSecRwLtStHdrstFrwdBkwdPosMax_180_Val/1 -> Bus Creator5/8  "HdrstFrwdBkwdnwdPosMax"
  PA_KeSMSw4sVIPMDSecRwLtStHdrstFrwdBkwdPos_180_Val/1 -> Bus Creator5/7  "HdrstFrwdBkwdnwdPos"
  Bus Creator5/1 -> Multiport Switch/7  "VIP4sLAdpt"
  PA_KeSMSw4sVIPMDSecRwLtStLgrstOtwdInwdPos_Over180_Val/1 -> Bus Creator6/4  "LgrstOtwdInwdPos"
  PA_KeSMSw4sVIPMDSecRwLtStLgrstOtwdInwdPosMin_Over180_Val/1 -> Bus Creator6/6  "LgrstOtwdInwdPosMin"
  PA_KeSMSw4sVIPMDSecRwLtStHdrstUpwdDnwdPos_Over180_Val/1 -> Bus Creator6/1  "HdrstUpwdDnwdPos"
  PA_KeSMSw4sVIPMDSecRwLtStHdrstUpwdDnwdPosMin_Over180_Val/1 -> Bus Creator6/3  "HdrstUpwdDnwdPosMin"
  PA_KeSMSw4sVIPMDSecRwLtStHdrstUpwdDnwdPosMax_Over180_Val/1 -> Bus Creator6/2  "HdrstUpwdDnwdPosMax"
  PA_KeSMSw4sVIPMDSecRwLtStLgrstOtwdInwdPosMin_180_Val/1 -> Bus Creator6/5  "LgrstOtwdInwdPosMax"
  PA_KeSMSw4sVIPMDSecRwLtStHdrstFrwdBkwdPosMin_Over180_Val/1 -> Bus Creator6/9  "HdrstFrwdBkwdnwdPosMin"
  PA_KeSMSw4sVIPMDSecRwLtStHdrstFrwdBkwdPosMax_Over180_Val/1 -> Bus Creator6/8  "HdrstFrwdBkwdnwdPosMax"
  PA_KeSMSw4sVIPMDSecRwLtStHdrstFrwdBkwdPos_Over180_Val/1 -> Bus Creator6/7  "HdrstFrwdBkwdnwdPos"
  Bus Creator6/1 -> Multiport Switch/8  "VIP4sLAdpt"
  Bus Selector8/5 -> [K_HdrstFrwdBkwdnwdPosMax]  "<HdrstFrwdBkwdnwdPosMax>"
  Bus Selector8/6 -> [K_HdrstFrwdBkwdnwdPosMin]  "<HdrstFrwdBkwdnwdPosMin>"
  PosDeltaCalib/1 -> Bus Selector9/1
  Bus Selector9/3 -> [KeSMSuSecRwStLegrestInOutPosDelta_Val]  "<KeSMSuSecRwStLegrestInOutPosDelta_Val>"
  Bus Selector9/6 -> [KeSMSuSecRwStLegrestUpwdDwnwdPosDelta_Val]  "<KeSMSuSecRwStLegrestUpwdDwnwdPosDelta_Val>"
  Bus Selector9/2 -> [KeSMSuSecRwStHeadrestUpwdDwnwdPosDelta_Val]  "<KeSMSuSecRwStHeadrestUpwdDwnwdPosDelta_Val>"
  Bus Selector9/4 -> [KeSMSuSecRwStFtrstUpwdDnwdPosDelta_Val]  "<KeSMSuSecRwStFtrstUpwdDnwdPosDelta_Val>"
  Bus Selector9/1 -> [KeSMSuSecRwStHeadrestFwdBkwdPosDelta_Val]  "<KeSMSuSecRwStHeadrestFwdBkwdPosDelta_Val>"
  Bus Selector9/5 -> [KeSMSuSecRwStBackPosDelta_Val]  "<KeSMSuSecRwStBackPosDelta_Val>"
